simulink model "CTADP_Demo"  (Simulink 7.5)
settings: Solver=ode45  StartTime=0.0  StopTime=10  FixedStep=0.01  MaxStep=0.01  RelTol=1e-3
libraries: CTADP_lib x1
settings Model: Creator=Yuri  LastModifiedBy=Yuri
settings SolverCC: ZeroCrossControl=EnableAll  ZeroCrossAlgorithm=Adaptive
settings OptimizationCC: ExpressionDepthLimit=128
settings DebuggingCC: UnderspecifiedInitializationDetection=Simplified  MergeDetectMultiDrivingBlocksExec=error  MultiTaskDSMMsg=none  FcnCallInpInsideContextMsg=Enable All  StateNameClashWarn=none
settings CodeAppCC: CustomSymbolStrType=$N$R$M_T
settings GRTTargetCC: TargetFunctionLibrary=C89/C90 (ANSI)

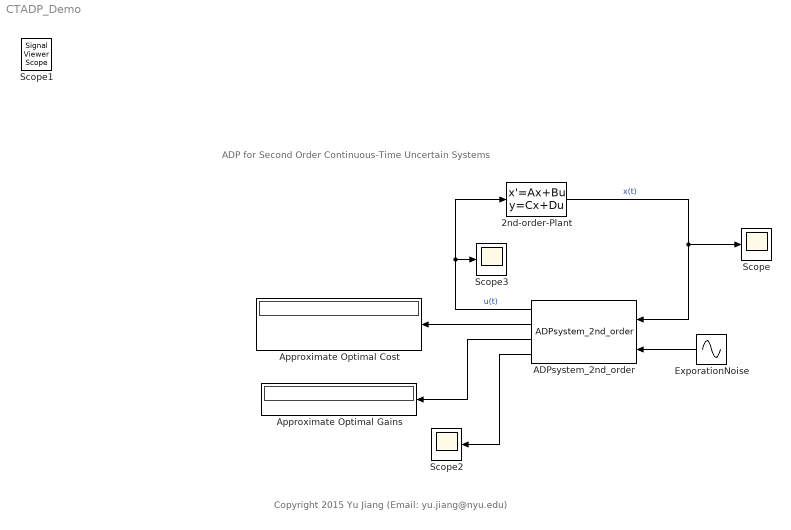
== system CTADP_Demo ==
  note: ADP for Second Order Continuous-Time Uncertain Systems
  note: Copyright 2015 Yu Jiang (Email: yu.jiang@nyu.edu)
  2nd-order-Plant : StateSpace  A=[0 1;-0.2 -0.1];  B=[0.03;.6];  C=eye(2);  D=zeros(2,1);  X0=[1;2]
  ADPsystem_2nd_order : CTADP_lib/ADPsystem_2nd_order  K=[0,0]  Q=eye(2)  R=1  dT=0.1
  Approximate Optimal Cost : Display
  Approximate Optimal Gains : Display
  "ExporationNoise " : Sin  Amplitude=0.1  Frequency=10  SampleTime=0
  Scope : Scope
      settings: SaveName=ADPresults
  Scope2 : Scope
      settings: SaveName=ScopeData3
  Scope3 : Scope
  Scope1 : SignalViewerScope  IOType=viewer  SampleTime=0
      settings: SaveName=ScopeData2  DataFormat=StructureWithTime
  wires:
  2nd-order-Plant/1 -> ADPsystem_2nd_order/1, Scope/1  "x(t)"
  ADPsystem_2nd_order/1 -> 2nd-order-Plant/1, Scope3/1  "u(t)"
  "ExporationNoise "/1 -> ADPsystem_2nd_order/2
  ADPsystem_2nd_order/2 -> Approximate Optimal Cost/1
  ADPsystem_2nd_order/3 -> Approximate Optimal Gains/1
  ADPsystem_2nd_order/4 -> Scope2/1
